simulink model "Problema3"  (R2016a)
settings: Solver=VariableStepDiscrete  StartTime=0.0  StopTime=20  RelTol=1e-3
undefined symbols (not defined in the file): m, n
settings Model: Creator=Cristina  LastModifiedBy=Cristina

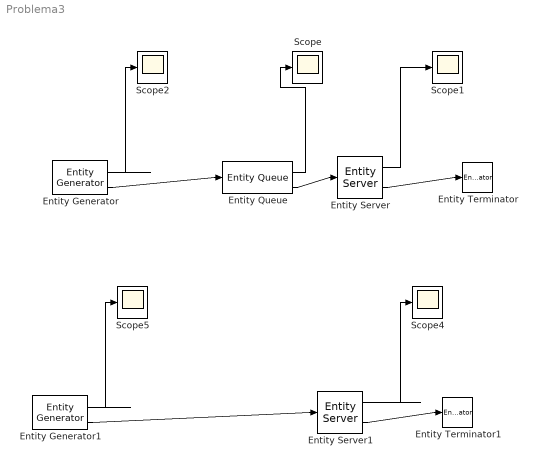
== system Problema3 ==
  Entity Generator : EntityGenerator  OutputPortMessageModes=n,m  IntergenerationTimeAction=dt = 1;  NumberEntitiesDeparted=on  EntityType=Structured  EntityTypeName=Entity
      settings: OutputPortMap=o0,o3
  Entity Generator1 : EntityGenerator  OutputPortMessageModes=n,m  IntergenerationTimeAction=dt = 1;  NumberEntitiesDeparted=on  EntityType=Structured  EntityTypeName=Entity
      settings: OutputPortMap=o0,o3
  Entity Queue : EntityQueue  InputPortMessageModes=m  OutputPortMessageModes=n,m  NumberEntitiesInBlock=on
      settings: OutputPortMap=o1,o5
  Entity Server : EntityServer  InputPortMessageModes=m  OutputPortMessageModes=n,m  Capacity=1  ServiceTimeValue=1.2  ServiceTimeAction=dt = 0.8 + 0.4*rand;  NumberEntitiesDeparted=on
      settings: OutputPortMap=o0,o9
  Entity Server1 : EntityServer  InputPortMessageModes=m  OutputPortMessageModes=n,m  Capacity=1  ServiceTimeValue=1.2  ServiceTimeAction=dt = 0.8 + 0.4*rand;  NumberEntitiesDeparted=on
      settings: OutputPortMap=o0,o9
  Entity Terminator : EntityTerminator  InputPortMessageModes=m
  Entity Terminator1 : EntityTerminator  InputPortMessageModes=m
  Scope{,1..2,4..5} (5 alike) : Scope
  wires:
  Entity Generator/2 -> Entity Queue/1
  Entity Queue/2 -> Entity Server/1
  Entity Server/2 -> Entity Terminator/1
  Entity Queue/1 -> Scope/1
  Entity Server/1 -> Scope1/1
  Entity Generator/1 -> Scope2/1
  Entity Generator1/2 -> Entity Server1/1
  Entity Server1/2 -> Entity Terminator1/1
  Entity Server1/1 -> Scope4/1
  Entity Generator1/1 -> Scope5/1
